simulink model "PostSubmission_FreqResp_00"  (R2018a)
settings: Solver=VariableStepAuto  StartTime=0.0  StopTime=Ttot  RelTol=1e-3
values from neighbouring files (symbols this model uses):
  f_LPF_noise = 1000    [Basics_01_Param.m]    (also in PostSubmission_FreqResp_00_Param.m)
  fn = 60    [Basics_01_Param.m]    (also in FIRs.m = 50; PostSubmission_FreqResp_00_Param.m; XoverRCalc.m)
  ImpulseAmp = 1    [PostSubmission_FreqResp_00_Param.m]
  ImpulseTime = 1 / (10*fn)    (= 0.00166666666667)    [PostSubmission_FreqResp_00_Param.m]
  L = X / 2 / pi / fn    (= 0.00132629119243)    [Basics_01_Param.m]    (also in PostSubmission_FreqResp_00_Param.m)
  Pos_1_Neg_minus1 = 1    [PostSubmission_FreqResp_00_Param.m]
  R = X/20    (= 0.025)    [Basics_01_Param.m]    (also in PostSubmission_FreqResp_00_Param.m)
  Ts_control = 1/20000    (= 5e-05)    [Basics_01_Param.m]    (also in PostSubmission_FreqResp_00_Param.m)
  zeta = 1    [Basics_01_Param.m]    (also in PostSubmission_FreqResp_00_Param.m)
libraries: PhD_Library x7, powerlib_meascontrol x7, powerlib x6, simulink x1
settings Model: SimulationMode=accelerator  Creator=daniemot  LastModifiedBy=daniemot
settings SolverCC: AutoInsertRateTranBlk=on
settings DataIOCC: ExternalInput=getinputstruct(WN_50mF_op_snapshot1)  InitialState=getstatestruct(WN_50mF_op_snapshot1)  SaveFinalState=on  SaveFormat=StructureWithTime  SaveOutput=off  SignalLogging=off  DSMLogging=off  SaveTime=off
settings DebuggingCC: ReadBeforeWriteMsg=DisableAll  WriteAfterWriteMsg=DisableAll  WriteAfterReadMsg=DisableAll  MultiTaskDSMMsg=none
settings ModelReferenceCC: UpdateModelReferenceTargets=IfOutOfDate
settings SFSimCC: SFSimEcho=off

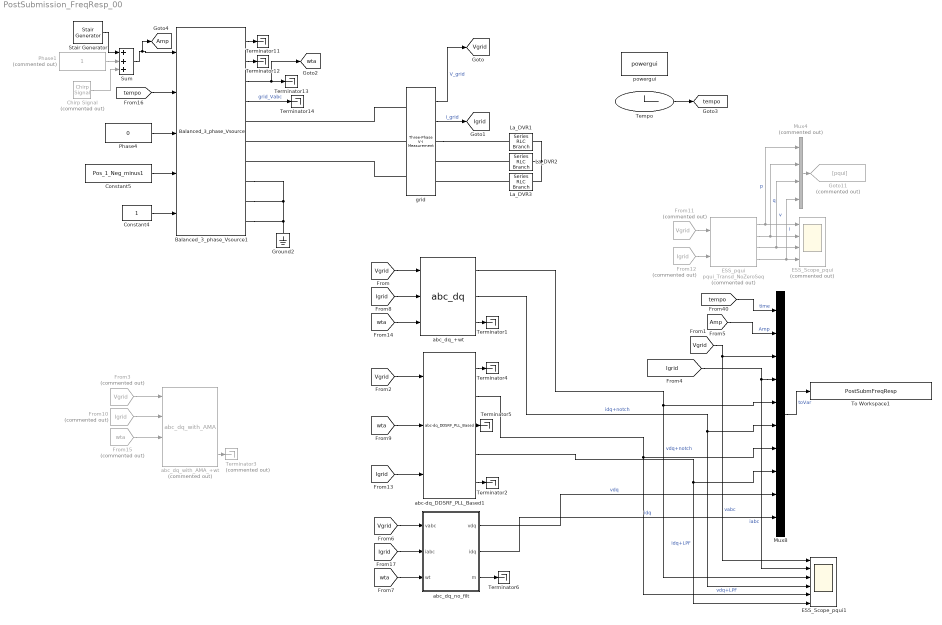
== system PostSubmission_FreqResp_00 ==
  Balanced_3_phase_Vsource1 : PhD_Library/Offshore_Oil_and_Wind/Balanced_3_phase_Vsource  BaseAmp=Uanp  fn=fn
  Chirp Signal : simulink/Sources/Chirp Signal  Commented=on  f1=0.1  T=9.8  f2=120
  Constant4 : Constant
  Constant5 : Constant  Value=Pos_1_Neg_minus1
  ESS_Scope_pqui : Scope  Commented=on  NumInputPorts=4
  ESS_Scope_pqui1 : Scope  NumInputPorts=6
  ESS_pqui : PhD_Library/Offshore_Oil_and_Wind/pqui_Transd_NoZeroSeq  Commented=on  Sn=3/2  Uanp=1  Iap=1
  From10 : From  Commented=on  GotoTag=Igrid  TagVisibility=global
  From11 : From  Commented=on  GotoTag=Vgrid  TagVisibility=global
  From12 : From  Commented=on  GotoTag=Igrid  TagVisibility=global
  From15 : From  Commented=on  GotoTag=wta  TagVisibility=global
  From3 : From  Commented=on  GotoTag=Vgrid  TagVisibility=global
  Goto11 : Goto  Commented=on  GotoTag=pqui
  Ground2 : powerlib/Elements/Ground  LConnTagsString=a
  La_DVR1 : powerlib/Elements/Series RLC Branch  LConnTagsString=__new0  RConnTagsString=__new0  BranchType=RL  Resistance=R  Inductance=L  SetiL0=off  InitialCurrent=0  Capacitance=1.0  Setx0=off  InitialVoltage=0  Measurements=None
  La_DVR2 : powerlib/Elements/Series RLC Branch  LConnTagsString=__new0  RConnTagsString=__new0  BranchType=RL  Resistance=R  Inductance=L  SetiL0=off  InitialCurrent=0  Capacitance=1.0  Setx0=off  InitialVoltage=0  Measurements=None
  La_DVR3 : powerlib/Elements/Series RLC Branch  LConnTagsString=__new0  RConnTagsString=__new0  BranchType=RL  Resistance=R  Inductance=L  SetiL0=off  InitialCurrent=0  Capacitance=1.0  Setx0=off  InitialVoltage=0  Measurements=None
  Mux4 : Mux  Commented=on
  Mux8 : Mux  Inputs=10
  Phase1 : Constant  Commented=on
  Phase4 : Constant  Value=0
  Stair Generator : powerlib_meascontrol/Pulse & Signal Generators/Stair Generator  t=[0 ImpulseTime]  e=[ImpulseAmp 0]  Ts=0
      settings: SourceProductName=Simscape Power Systems
  Sum : Sum  Inputs=+++
  Tempo : Clock
  Terminator{1..2,4..6,11..14} (9 alike) : Terminator
  Terminator3 : Terminator  Commented=on
  To Workspace1 : ToWorkspace  VariableName=PostSubmFreqResp  SampleTime=Ts_control
  abc-dq_DDSRF_PLL_Based1 : PhD_Library/Offshore_Oil_and_Wind/abc-dq_DDSRF_PLL_Based  Ts=Ts_control  fc=fn/2^0.5
  abc_dq_+wt : PhD_Library/Offshore_Oil_and_Wind/abc_dq  Ts=Ts_control  fn=2*fn  fcutoutv=f_LPF_noise  fcutouti=f_LPF_noise  zeta=zeta
      link override Second-Order Filter2: PlotResponse=off
  abc_dq_no_filt : Subsystem  mask(abc->dq with Matlab){Ts=Ts_control, fn=2*fn, fcutoutv=f_LPF_noise, fcutouti=f_LPF_noise, zeta=zeta}
      mask prompts: Ts "Sampling time [s]"; fn "Notch frequency [Hz]"; fcutoutv "Cutout freq. low-pass for vdq meas. [Hz]"; fcutouti "Cutout freq. low-pass for idq meas. [Hz]"; zeta "Zeta for notch filters"
  abc_dq_with_AMA_+wt : PhD_Library/Offshore_Oil_and_Wind/abc_dq_with_AMA  Commented=on  Ts=Ts_control  fn=fn  fmin=fn*0.8  fmax=fn*1.2  fcutoutv=f_LPF_noise  fcutouti=f_LPF_noise
  grid : powerlib/Measurements/Three-Phase V-I Measurement  VoltageMeasurement=phase-to-ground  SetLabelV=off  LabelV=vconv  Vpu=off  VpuLL=off  CurrentMeasurement=yes  SetLabelI=off  LabelI=iconv  Ipu=off  Pbase=sn  Vbase=uab  OutputType=Complex  PhasorSimulation=off  PSBequivalent=0
  powergui : powerlib/powergui  Priority=1  SimulationMode=Discrete  SampleTime=5e-6  frequency=60  Iterations=50  frequencyindice=0  Pbase=100e6  ErrMax=1e-4  UnitsV=kV  UnitsW=MW  buscounter=0  FunctionMessages=off  echomessages=off  EnableUseOfTLC=off  CurrentSourceSwitches=off  DisableSnubberDevices=off  DisableRonSwitches=off  DisableVfSwitches=off  DisplayEquations=off  SolverType=Tustin/Backward Euler (TBE)  Interpol=off  ExternalGateDelay=off  methode=off  Ts=100  x0status=blocks  SPID=off  SwTol=0  HookPort=off  RestoreLinks=warning  ResistiveCurrentMeasurement=off  Frange=[0:2:500]  Ylog=off  Xlog=on  ShowGrid=off  save=off  variable=ZData  structure=0  ZoomFFT=off  StartTime=0.0  cycles=1  DisplayStyle=1  fundamental=60  FreqAxis=off  MaxFrequency=1000  frequencyindicesteady=1  RmsSteady=1  display=off
  tag scope: Amp=global, Igrid=global, Vgrid=global, tempo=global, wta=global
  wires:
  ESS_pqui/3 -> Mux4/3, ESS_Scope_pqui/3  "v"
  ESS_pqui/2 -> Mux4/2, ESS_Scope_pqui/2  "q"
  ESS_pqui/4 -> Mux4/4, ESS_Scope_pqui/4  "i"
  ESS_pqui/1 -> Mux4/1, ESS_Scope_pqui/1  "p"
  grid/1 -> [Vgrid]  "V_grid"
  grid/2 -> [Igrid]  "I_grid"
  Tempo/1 -> [tempo]
  Sum/1 -> Balanced_3_phase_Vsource1/1, [Amp]
  Phase4/1 -> Balanced_3_phase_Vsource1/3
  [tempo] -> Balanced_3_phase_Vsource1/2
  Constant4/1 -> Balanced_3_phase_Vsource1/5
  Constant5/1 -> Balanced_3_phase_Vsource1/4
  Balanced_3_phase_Vsource1/1 -> Terminator11/1
  Balanced_3_phase_Vsource1/2 -> Terminator12/1
  Balanced_3_phase_Vsource1/4 -> Terminator14/1  "grid_Vabc"
  From11/1 -> ESS_pqui/1
  From12/1 -> ESS_pqui/2
  Mux8/1 -> To Workspace1/1  "toVar"
  [tempo] -> Mux8/1  "time"
  [Vgrid] -> ESS_Scope_pqui1/1, Mux8/3  "vabc"
  [Igrid] -> Mux8/4, ESS_Scope_pqui1/2  "iabc"
  abc_dq_+wt/1 -> ESS_Scope_pqui1/3, Mux8/5  "vdq+notch"
  Mux4/1 -> Goto11/1
  abc_dq_+wt/2 -> ESS_Scope_pqui1/4, Mux8/6  "idq+notch"
  [Vgrid] -> abc_dq_+wt/1
  [Vgrid] -> abc-dq_DDSRF_PLL_Based1/1
  From3/1 -> abc_dq_with_AMA_+wt/1
  [Igrid] -> abc_dq_+wt/2
  [wta] -> abc-dq_DDSRF_PLL_Based1/2
  From10/1 -> abc_dq_with_AMA_+wt/2
  [Igrid] -> abc-dq_DDSRF_PLL_Based1/3
  [wta] -> abc_dq_+wt/3
  From15/1 -> abc_dq_with_AMA_+wt/3
  abc_dq_+wt/3 -> Terminator1/1
  abc-dq_DDSRF_PLL_Based1/5 -> Terminator2/1
  abc_dq_with_AMA_+wt/3 -> Terminator3/1
  abc-dq_DDSRF_PLL_Based1/2 -> ESS_Scope_pqui1/5, Mux8/7  "vdq+LPF"
  abc-dq_DDSRF_PLL_Based1/4 -> ESS_Scope_pqui1/6, Mux8/8  "idq+LPF"
  abc-dq_DDSRF_PLL_Based1/1 -> Terminator4/1
  abc-dq_DDSRF_PLL_Based1/3 -> Terminator5/1
  Balanced_3_phase_Vsource1/3 -> [wta], Terminator13/1
  [Amp] -> Mux8/2  "Amp"
  Stair Generator/1 -> Sum/1
  Phase1/1 -> Sum/2
  Chirp Signal/1 -> Sum/3
  [wta] -> abc_dq_no_filt/3(wt)
  [Vgrid] -> abc_dq_no_filt/1(vabc)
  [Igrid] -> abc_dq_no_filt/2(iabc)
  abc_dq_no_filt/1(vdq) -> Mux8/9  "vdq"
  abc_dq_no_filt/2(idq) -> Mux8/10  "idq"
  abc_dq_no_filt/3(m) -> Terminator6/1
  connections:
  grid/RConn1 -- La_DVR1/RConn1
  La_DVR2/RConn1 -- grid/RConn2
  La_DVR3/RConn1 -- grid/RConn3
  La_DVR1/LConn1 -- La_DVR3/LConn1 -- La_DVR2/LConn1
  Balanced_3_phase_Vsource1/RConn4 -- Balanced_3_phase_Vsource1/RConn5 -- Balanced_3_phase_Vsource1/RConn6 -- Ground2/LConn1
  grid/LConn1 -- Balanced_3_phase_Vsource1/RConn1
  grid/LConn2 -- Balanced_3_phase_Vsource1/RConn2
  grid/LConn3 -- Balanced_3_phase_Vsource1/RConn3

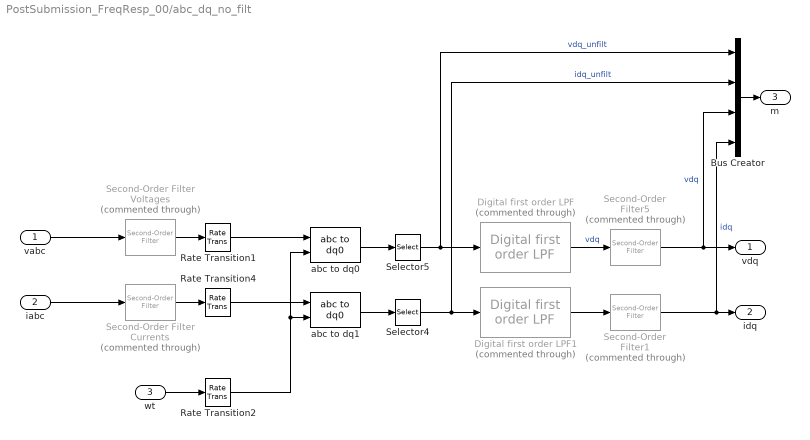
== system PostSubmission_FreqResp_00/abc_dq_no_filt ==
  vabc : Inport
  iabc : Inport  Port=2
  wt : Inport  Port=3
  Bus Creator : BusCreator  Inputs=4
  Digital first order LPF : PhD_Library/Offshore_Oil_and_Wind/Digital first order LPF  Commented=through  Ts=Ts  fcutout=fcutoutv
  Digital first order LPF1 : PhD_Library/Offshore_Oil_and_Wind/Digital first order LPF  Commented=through  Ts=Ts  fcutout=fcutouti
  Rate Transition1 : RateTransition  OutPortSampleTime=Ts
  Rate Transition2 : RateTransition  OutPortSampleTime=Ts
  Rate Transition4 : RateTransition  OutPortSampleTime=Ts
  Second-Order Filter1 : powerlib_meascontrol/Filters/Second-Order Filter  Commented=through  FilterType=Bandstop (Notch)  Fo=fn  Zeta=zeta  Ts=Ts  Initialize=off  Vac_Init="[0,  0,  60]"  Vdc_Init=0  PlotResponse=off  FreqRange=[0, 1000, 0.1]
      settings: SourceProductName=Simscape Power Systems  SourceProductBaseCode=PS
  Second-Order Filter5 : powerlib_meascontrol/Filters/Second-Order Filter  Commented=through  FilterType=Bandstop (Notch)  Fo=fn  Zeta=zeta  Ts=Ts  Initialize=off  Vac_Init="[0,  0,  60]"  Vdc_Init=0  PlotResponse=off  FreqRange=[0, 1000, 0.1]
      settings: SourceProductName=Simscape Power Systems  SourceProductBaseCode=PS
  Second-Order Filter Currents : powerlib_meascontrol/Filters/Second-Order Filter  Commented=through  FilterType=Lowpass  Fo=fcutoutv  Zeta=zeta  Ts=Ts  Initialize=off  Vac_Init="[0,  0,  60]"  Vdc_Init=0  PlotResponse=off  FreqRange=[0, 1000, 0.1]
      settings: SourceProductName=Simscape Power Systems  SourceProductBaseCode=PS
  Second-Order Filter Voltages : powerlib_meascontrol/Filters/Second-Order Filter  Commented=through  FilterType=Lowpass  Fo=fcutoutv  Zeta=zeta  Ts=0  Initialize=off  Vac_Init="[0,  0,  60]"  Vdc_Init=0  PlotResponse=off  FreqRange=[0, 1000, 0.1]
      settings: SourceProductName=Simscape Power Systems  SourceProductBaseCode=PS
  Selector4 : Selector  InputPortWidth=3  IndexOptions=Index vector (dialog)  Indices=[1 2]  OutputSizes=1
  Selector5 : Selector  InputPortWidth=3  IndexOptions=Index vector (dialog)  Indices=[1 2]  OutputSizes=1
  abc to dq0 : powerlib_meascontrol/Transformations/abc to dq0  Alignment=90 degrees behind phase A axis
  abc to dq1 : powerlib_meascontrol/Transformations/abc to dq0  Alignment=90 degrees behind phase A axis
  vdq : Outport
  idq : Outport  Port=2
  m : Outport  Port=3
  wires:
  Second-Order Filter Currents/1 -> Rate Transition4/1
  Second-Order Filter Voltages/1 -> Rate Transition1/1
  vabc/1 -> Second-Order Filter Voltages/1
  wt/1 -> Rate Transition2/1
  Second-Order Filter5/1 -> Bus Creator/3, vdq/1  "vdq"
  Bus Creator/1 -> m/1
  abc to dq0/1 -> Selector5/1
  Rate Transition4/1 -> abc to dq1/1
  Selector4/1 -> Digital first order LPF1/1, Bus Creator/2  "idq_unfilt"
  Rate Transition2/1 -> abc to dq0/2, abc to dq1/2
  iabc/1 -> Second-Order Filter Currents/1
  Rate Transition1/1 -> abc to dq0/1
  Selector5/1 -> Bus Creator/1, Digital first order LPF/1  "vdq_unfilt"
  Second-Order Filter1/1 -> idq/1, Bus Creator/4  "idq"
  abc to dq1/1 -> Selector4/1
  Digital first order LPF/1 -> Second-Order Filter5/1  "vdq"
  Digital first order LPF1/1 -> Second-Order Filter1/1
